simulink model "gm_sampleModel1762_5_sub"  (R2023a)
settings: Solver=VariableStepAuto  StartTime=0.0  StopTime=10.0  RelTol=1e-3
settings Model: Creator=user1  LastModifiedBy=user1
settings OptimizationCC: BlockReduction=off  ConditionallyExecuteInputs=off
settings DebuggingCC: InheritedTsInSrcMsg=none

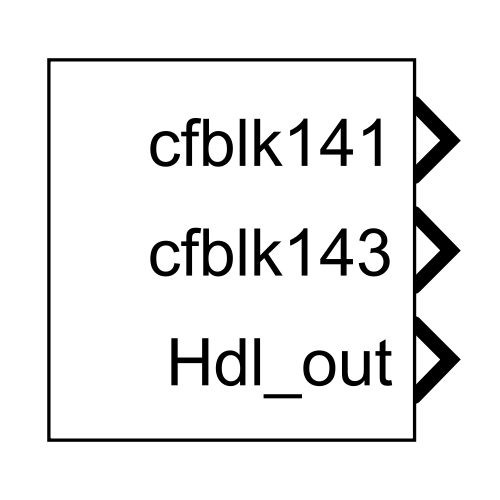
[thumbnail: Simulink's stored preview of the top-level diagram]
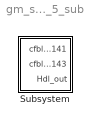
== system gm_sampleModel1762_5_sub ==
  Subsystem : Subsystem

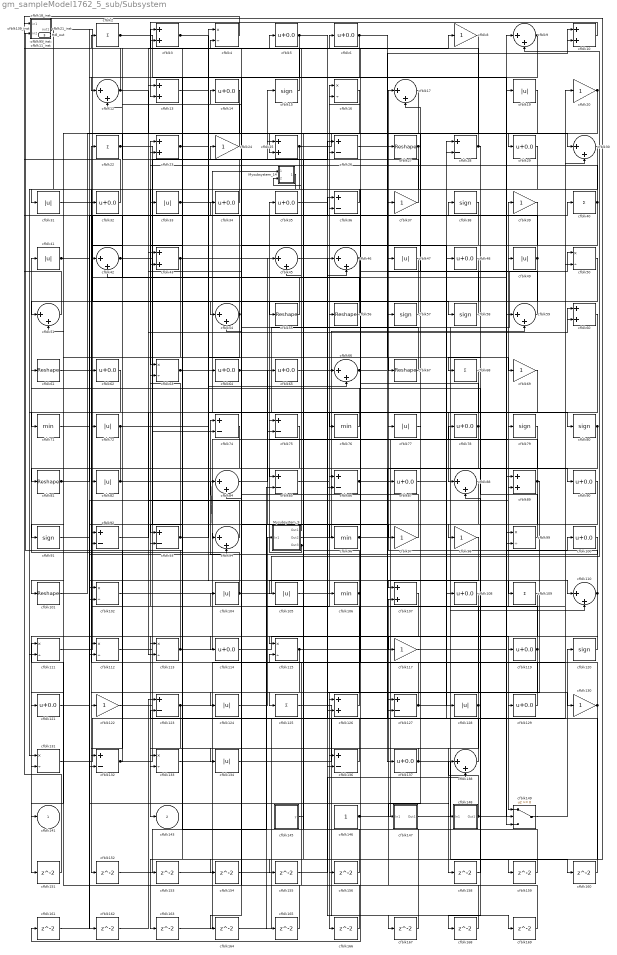
== system gm_sampleModel1762_5_sub/Subsystem ==
  Mysubsystem_14 : Subsystem
  Mysubsystem_9 : Subsystem
  cfblk{3,10,13,23,25,43,60,89,107,126} (10 alike) : Sum  OutDataTypeStr=uint8
  cfblk{5..6,14,29,32,34..35,48,62,64..65,78,87,90,100,108,114,119,121,129,137} (21 alike) : Bias  Bias=0.0  SaturateOnIntegerOverflow=off
  cfblk{27,55..56,61,67,81,101} (7 alike) : Reshape
  cfblk{4,16,50,63,99,102,111..113,115,131,133} (12 alike) : Product  Inputs=*/  OutDataTypeStr=uint8  RndMeth=Zero  SaturateOnIntegerOverflow=on
  cfblk103_inst : Subsystem
  cfblk{19,31,33,41,47,49,72,77,82,104..105,124,128,134} (14 alike) : Abs  OutDataTypeStr=uint8  SaturateOnIntegerOverflow=off
  cfblk{71,76,96,106} (4 alike) : MinMax  OutDataTypeStr=uint8
  cfblk{2,22,40,68,109,125} (6 alike) : Sum  Inputs=+  OutDataTypeStr=uint8
  cfblk{9,12,17,30,42,45..46,51,54,59,66,84,88,94,110,138} (16 alike) : Sum  Inputs=|++  OutDataTypeStr=uint8
  cfblk{8,20,24,37,39,69,97..98,117,122,130} (11 alike) : Gain  OutDataTypeStr=uint8
  cfblk11_inst : Subsystem
  cfblk{15,38,57..58,79..80,91,120} (8 alike) : Signum
  cfblk{26,28,36,74..75,85..86,92..93,123,127,132,136} (13 alike) : Sum  Inputs=+-  OutDataTypeStr=uint8
  cfblk139_inst : Subsystem
  cfblk145 : Subsystem  mask(Counter Free-Running){NumBits=double(16), tsamp=double(-1)}
      mask prompts: NumBits "Simulink:masks:NumberOfBits_MP"; tsamp "Simulink:masks:SampleTime_MP"
      mask help: Simulink:masks:CounterFreeRunning_MD
  cfblk146 : Constant  OutDataTypeStr=uint8  SampleTime=-1
  cfblk147 : Subsystem
  cfblk148 : Subsystem
  cfblk149 : Switch  OutDataTypeStr=uint8  SaturateOnIntegerOverflow=off  InputSameDT=off
  cfblk{151..156,158..169} (18 alike) : Delay  SampleTime=1
  cfblk18_inst : Subsystem
  cfblk21_inst : Subsystem
  cfblk95_inst : Subsystem
  cfblk141 : Outport  OutDataTypeStr=uint8  SampleTime=1  VectorParamsAs1DForOutWhenUnconnected=off
  cfblk143 : Outport  Port=2  OutDataTypeStr=uint8  SampleTime=1  VectorParamsAs1DForOutWhenUnconnected=off
  Hdl_out : Outport  Port=3  OutDataTypeStr=uint8  SampleTime=1
  wires:
  Mysubsystem_14/1(Out1) -> cfblk152/1
  Mysubsystem_9/1(Out1) -> cfblk45/2
  Mysubsystem_9/2(Out2) -> cfblk59/2
  Mysubsystem_9/3(Out3) -> cfblk4/2, cfblk24/1
  cfblk10/1 -> cfblk13/2
  cfblk100/1 -> cfblk74/1
  cfblk101/1 -> cfblk25/2
  cfblk102/1 -> cfblk17/1
  cfblk103_inst/1(out1) -> cfblk58/1, Hdl_out/1
  cfblk104/1 -> cfblk9/2, cfblk84/2, cfblk41/1
  cfblk105/1 -> cfblk16/1
  cfblk106/1 -> cfblk42/2, cfblk166/1
  cfblk107/1 -> cfblk143/1
  cfblk108/1 -> cfblk161/1
  cfblk109/1 -> cfblk149/1
  cfblk11_inst/1(out1) -> cfblk159/1
  cfblk110/1 -> cfblk77/1, cfblk151/1, cfblk131/2
  cfblk111/1 -> cfblk35/1
  cfblk112/1 -> cfblk74/2
  cfblk113/1 -> cfblk36/2, cfblk139_inst/2(in2)
  cfblk114/1 -> cfblk119/1
  cfblk115/1 -> cfblk28/2, cfblk122/1
  cfblk117/1 -> cfblk19/1
  cfblk119/1 -> cfblk23/1, cfblk126/1, cfblk39/1, cfblk125/1
  cfblk12/1 -> cfblk95_inst/1(in1), cfblk30/1
  cfblk120/1 -> cfblk114/1
  cfblk121/1 -> cfblk89/2
  cfblk122/1 -> cfblk37/1
  cfblk123/1 -> cfblk48/1, cfblk133/2
  cfblk124/1 -> cfblk106/1
  cfblk125/1 -> cfblk167/1
  cfblk126/1 -> cfblk22/1
  cfblk127/1 -> cfblk92/1, cfblk50/1
  cfblk128/1 -> cfblk158/1, cfblk156/1, Mysubsystem_9/1(In1)
  cfblk129/1 -> cfblk14/1
  cfblk13/1 -> cfblk110/1
  cfblk130/1 -> cfblk163/1, cfblk16/2
  cfblk131/1 -> cfblk107/2
  cfblk132/1 -> cfblk92/2, cfblk87/1, cfblk38/1
  cfblk133/1 -> cfblk57/1
  cfblk134/1 -> cfblk27/1
  cfblk136/1 -> cfblk123/2
  cfblk137/1 -> cfblk160/1, cfblk133/1
  cfblk138/1 -> cfblk104/1
  cfblk139_inst/1(out1) -> cfblk162/1
  cfblk14/1 -> cfblk51/2
  cfblk145/1(y) -> cfblk75/1
  cfblk146/1 -> cfblk59/1, cfblk20/1
  cfblk147/1(Out1) -> cfblk110/2
  cfblk148/1(Out1) -> cfblk138/1, cfblk100/1
  cfblk149/1 -> cfblk120/1
  cfblk15/1 -> cfblk5/1
  cfblk151/1 -> cfblk18_inst/2(in2)
  cfblk152/1 -> cfblk85/2
  cfblk153/1 -> cfblk50/2
  cfblk154/1 -> cfblk46/1
  cfblk155/1 -> cfblk138/2
  cfblk156/1 -> cfblk25/1
  cfblk158/1 -> cfblk88/2
  cfblk159/1 -> cfblk3/1
  cfblk16/1 -> cfblk132/1
  cfblk160/1 -> cfblk28/1
  cfblk161/1 -> cfblk102/1
  cfblk162/1 -> cfblk123/1
  cfblk163/1 -> cfblk99/2
  cfblk164/1 -> cfblk30/2
  cfblk165/1 -> cfblk54/2
  cfblk166/1 -> cfblk115/2
  cfblk167/1 -> cfblk93/2
  cfblk168/1 -> cfblk127/1
  cfblk169/1 -> cfblk111/1
  cfblk17/1 -> cfblk115/1
  cfblk18_inst/1(out1) -> cfblk66/1
  cfblk19/1 -> cfblk147/1(In1)
  cfblk2/1 -> cfblk89/1, cfblk6/1
  cfblk20/1 -> cfblk72/1, cfblk42/1
  cfblk21_inst/1(out1) -> cfblk131/1
  cfblk22/1 -> cfblk8/1, cfblk165/1
  cfblk23/1 -> cfblk66/2, cfblk76/1
  cfblk24/1 -> cfblk21_inst/1(in1)
  cfblk25/1 -> cfblk29/1, cfblk71/1
  cfblk26/1 -> cfblk69/1
  cfblk27/1 -> cfblk136/1, cfblk63/1
  cfblk28/1 -> cfblk95_inst/2(in2), cfblk68/1
  cfblk29/1 -> cfblk153/1
  cfblk3/1 -> cfblk67/1, cfblk45/1
  cfblk30/1 -> cfblk124/1
  cfblk31/1 -> cfblk108/1
  cfblk32/1 -> cfblk11_inst/2(in2)
  cfblk33/1 -> cfblk136/2, Mysubsystem_14/1(In1)
  cfblk34/1 -> cfblk2/1
  cfblk35/1 -> cfblk46/2
  cfblk36/1 -> cfblk31/1
  cfblk37/1 -> cfblk12/2
  cfblk38/1 -> cfblk155/1
  cfblk39/1 -> cfblk168/1
  cfblk4/1 -> cfblk139_inst/1(in1)
  cfblk40/1 -> cfblk23/2, cfblk126/2, cfblk164/1
  cfblk41/1 -> cfblk94/2, cfblk34/1
  cfblk42/1 -> cfblk15/1, cfblk40/1
  cfblk43/1 -> cfblk137/1, cfblk132/2
  cfblk45/1 -> cfblk80/1
  cfblk46/1 -> cfblk93/1, cfblk75/2
  cfblk47/1 -> cfblk121/1
  cfblk48/1 -> cfblk91/1
  cfblk49/1 -> cfblk54/1, cfblk26/2, cfblk103_inst/1(in1)
  cfblk5/1 -> cfblk130/1, cfblk113/1
  cfblk50/1 -> cfblk55/1
  cfblk51/1 -> cfblk21_inst/2(in2)
  cfblk54/1 -> cfblk103_inst/2(in2), cfblk101/1
  cfblk55/1 -> cfblk33/1
  cfblk56/1 -> cfblk32/1
  cfblk57/1 -> cfblk51/1
  cfblk58/1 -> cfblk17/2
  cfblk59/1 -> cfblk3/2
  cfblk6/1 -> cfblk47/1, cfblk12/1
  cfblk60/1 -> cfblk112/1
  cfblk61/1 -> cfblk9/1
  cfblk62/1 -> cfblk111/2
  cfblk63/1 -> cfblk149/2, cfblk99/1
  cfblk64/1 -> cfblk86/2, cfblk10/1
  cfblk65/1 -> cfblk169/1
  cfblk66/1 -> cfblk60/1, cfblk10/2
  cfblk67/1 -> cfblk11_inst/1(in1)
  cfblk68/1 -> cfblk88/1
  cfblk69/1 -> cfblk113/2
  cfblk71/1 -> cfblk62/1
  cfblk72/1 -> cfblk64/1, cfblk60/2, cfblk112/2
  cfblk74/1 -> cfblk141/1
  cfblk75/1 -> cfblk82/1
  cfblk76/1 -> cfblk4/1
  cfblk77/1 -> cfblk107/1
  cfblk78/1 -> cfblk18_inst/1(in1), cfblk127/2
  cfblk79/1 -> cfblk98/1
  cfblk8/1 -> cfblk43/2
  cfblk80/1 -> cfblk85/1, cfblk149/3
  cfblk81/1 -> cfblk36/1, cfblk109/1
  cfblk82/1 -> cfblk94/1, cfblk81/1
  cfblk84/1 -> cfblk65/1
  cfblk85/1 -> cfblk86/1
  cfblk86/1 -> cfblk90/1, cfblk78/1
  cfblk87/1 -> cfblk128/1
  cfblk88/1 -> cfblk105/1
  cfblk89/1 -> cfblk129/1, Mysubsystem_14/2(In2), cfblk96/1
  cfblk9/1 -> cfblk154/1, cfblk102/2
  cfblk90/1 -> cfblk134/1
  cfblk91/1 -> cfblk148/1(In1)
  cfblk92/1 -> cfblk56/1
  cfblk93/1 -> cfblk84/1, cfblk26/1, cfblk63/2
  cfblk94/1 -> cfblk13/1
  cfblk95_inst/1(out1) -> cfblk97/1
  cfblk96/1 -> cfblk79/1, cfblk49/1
  cfblk97/1 -> cfblk43/1
  cfblk98/1 -> cfblk117/1
  cfblk99/1 -> cfblk61/1

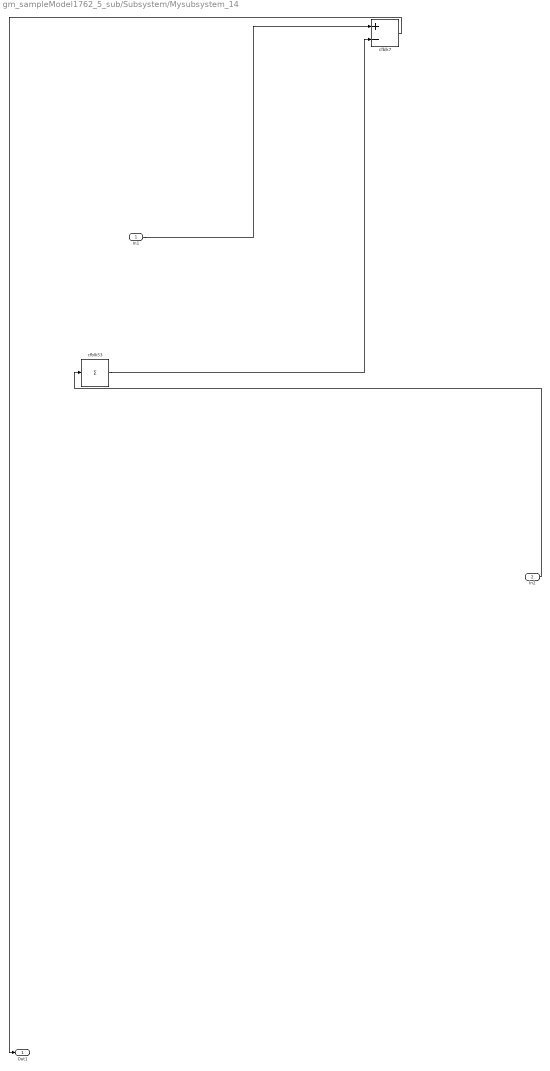
== system gm_sampleModel1762_5_sub/Subsystem/Mysubsystem_14 ==
  In1 : Inport  OutDataTypeStr=uint8  PortDimensions=1  SampleTime=1
  In2 : Inport  Port=2  OutDataTypeStr=uint8  PortDimensions=1  SampleTime=1
  cfblk53 : Sum  Inputs=+
  cfblk7 : Sum  Inputs=+-
  Out1 : Outport  SampleTime=1
  wires:
  In1/1 -> cfblk7/1
  In2/1 -> cfblk53/1
  cfblk53/1 -> cfblk7/2
  cfblk7/1 -> Out1/1

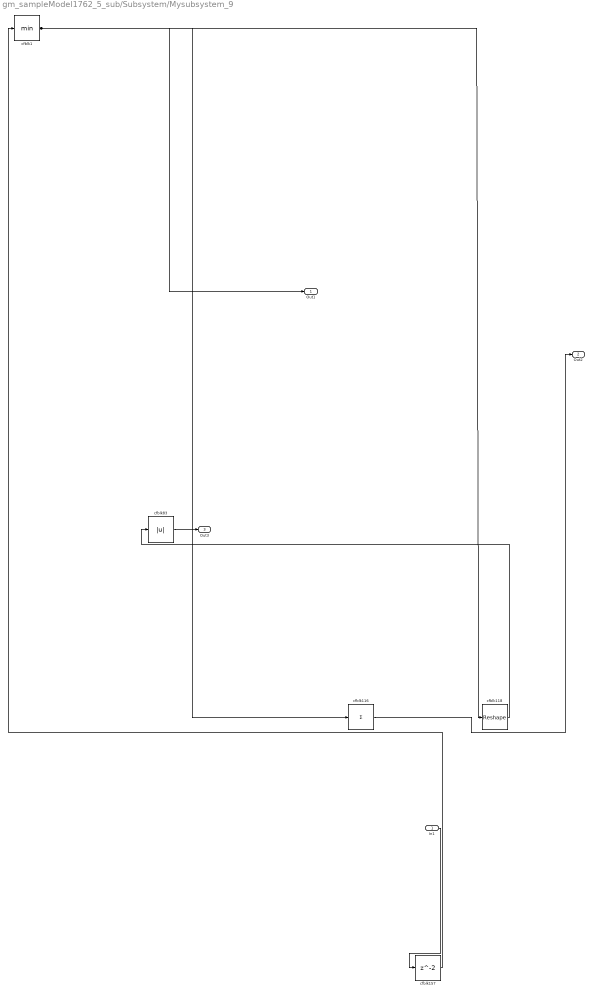
== system gm_sampleModel1762_5_sub/Subsystem/Mysubsystem_9 ==
  In1 : Inport  OutDataTypeStr=uint8  PortDimensions=1  SampleTime=1
  cfblk1 : MinMax
  cfblk116 : Sum  Inputs=+
  cfblk118 : Reshape
  cfblk157 : Delay  SampleTime=1
  cfblk83 : Abs  SaturateOnIntegerOverflow=off
  Out1 : Outport  SampleTime=1
  Out2 : Outport  Port=2  SampleTime=1
  Out3 : Outport  Port=3  SampleTime=1
  wires:
  In1/1 -> cfblk157/1
  cfblk1/1 -> cfblk118/1, Out1/1, cfblk116/1
  cfblk116/1 -> Out2/1
  cfblk118/1 -> cfblk83/1
  cfblk157/1 -> cfblk1/1
  cfblk83/1 -> Out3/1

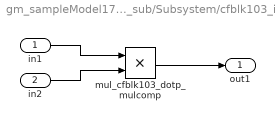
== system gm_sampleModel1762_5_sub/Subsystem/cfblk103_inst ==
  in1 : Inport  OutDataTypeStr=uint8  SampleTime=1
  in2 : Inport  Port=2  OutDataTypeStr=uint8  SampleTime=1
  mul_cfblk103_dotp_mulcomp : Product  Inputs=**  OutDataTypeStr=uint8  SampleTime=1
  out1 : Outport  OutDataTypeStr=uint8  SampleTime=1
  wires:
  in1/1 -> mul_cfblk103_dotp_mulcomp/1
  in2/1 -> mul_cfblk103_dotp_mulcomp/2
  mul_cfblk103_dotp_mulcomp/1 -> out1/1

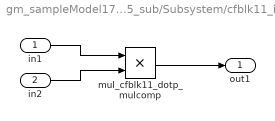
== system gm_sampleModel1762_5_sub/Subsystem/cfblk11_inst ==
  in1 : Inport  OutDataTypeStr=uint8  SampleTime=1
  in2 : Inport  Port=2  OutDataTypeStr=uint8  SampleTime=1
  mul_cfblk11_dotp_mulcomp : Product  Inputs=**  OutDataTypeStr=uint8  SampleTime=1
  out1 : Outport  OutDataTypeStr=uint8  SampleTime=1
  wires:
  in1/1 -> mul_cfblk11_dotp_mulcomp/1
  in2/1 -> mul_cfblk11_dotp_mulcomp/2
  mul_cfblk11_dotp_mulcomp/1 -> out1/1

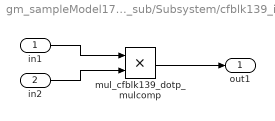
== system gm_sampleModel1762_5_sub/Subsystem/cfblk139_inst ==
  in1 : Inport  OutDataTypeStr=uint8  SampleTime=1
  in2 : Inport  Port=2  OutDataTypeStr=uint8  SampleTime=1
  mul_cfblk139_dotp_mulcomp : Product  Inputs=**  OutDataTypeStr=uint8  SampleTime=1
  out1 : Outport  OutDataTypeStr=uint8  SampleTime=1
  wires:
  in1/1 -> mul_cfblk139_dotp_mulcomp/1
  in2/1 -> mul_cfblk139_dotp_mulcomp/2
  mul_cfblk139_dotp_mulcomp/1 -> out1/1

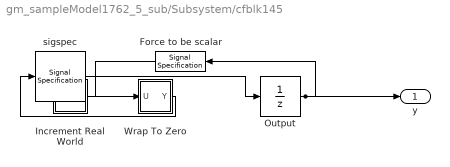
== system gm_sampleModel1762_5_sub/Subsystem/cfblk145 ==
  Force to be scalar : SignalSpecification  DisableCoverage=on  Dimensions=1
  Increment Real World : Subsystem  mask(Real World Value Increment){}
      mask help: Simulink:masks:RealWorldValueIncrement_MD
      mask Display: disp('V++')
  Output : UnitDelay  InitialCondition=0.0  SampleTime=tsamp  HasFrameUpgradeWarning=on
  Wrap To Zero : Subsystem  mask(Wrap To Zero){Threshold=double(65535)}
      mask prompts: Threshold "Simulink:masks:Threshold_MP"
      mask help: Simulink:masks:WrapToZero_MD
  sigspec : SignalSpecification  OutDataTypeStr=uint16  Dimensions=1
  y : Outport  SampleTime=1
  wires:
  Force to be scalar/1 -> Increment Real World/1(u)
  Increment Real World/1(y) -> Wrap To Zero/1(U)
  Output/1 -> Force to be scalar/1, y/1
  Wrap To Zero/1(Y) -> sigspec/1
  sigspec/1 -> Output/1

== system gm_sampleModel1762_5_sub/Subsystem/cfblk147 ==
  In1 : Inport  OutDataTypeStr=uint8  PortDimensions=1  SampleTime=1
  Out1 : Outport  SampleTime=1
  wires:
  In1/1 -> Out1/1

== system gm_sampleModel1762_5_sub/Subsystem/cfblk148 ==
  In1 : Inport  OutDataTypeStr=uint8  PortDimensions=1  SampleTime=1
  Out1 : Outport  SampleTime=1
  wires:
  In1/1 -> Out1/1

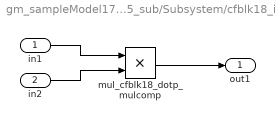
== system gm_sampleModel1762_5_sub/Subsystem/cfblk18_inst ==
  in1 : Inport  OutDataTypeStr=uint8  SampleTime=1
  in2 : Inport  Port=2  OutDataTypeStr=uint8  SampleTime=1
  mul_cfblk18_dotp_mulcomp : Product  Inputs=**  OutDataTypeStr=uint8  SampleTime=1
  out1 : Outport  OutDataTypeStr=uint8  SampleTime=1
  wires:
  in1/1 -> mul_cfblk18_dotp_mulcomp/1
  in2/1 -> mul_cfblk18_dotp_mulcomp/2
  mul_cfblk18_dotp_mulcomp/1 -> out1/1

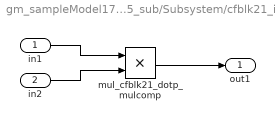
== system gm_sampleModel1762_5_sub/Subsystem/cfblk21_inst ==
  in1 : Inport  OutDataTypeStr=uint8  SampleTime=1
  in2 : Inport  Port=2  OutDataTypeStr=uint8  SampleTime=1
  mul_cfblk21_dotp_mulcomp : Product  Inputs=**  OutDataTypeStr=uint8  SampleTime=1
  out1 : Outport  OutDataTypeStr=uint8  SampleTime=1
  wires:
  in1/1 -> mul_cfblk21_dotp_mulcomp/1
  in2/1 -> mul_cfblk21_dotp_mulcomp/2
  mul_cfblk21_dotp_mulcomp/1 -> out1/1

== system gm_sampleModel1762_5_sub/Subsystem/cfblk95_inst ==
  in1 : Inport  OutDataTypeStr=uint8  SampleTime=1
  in2 : Inport  Port=2  OutDataTypeStr=uint8  SampleTime=1
  mul_cfblk95_dotp_mulcomp : Product  Inputs=**  OutDataTypeStr=uint8  SampleTime=1
  out1 : Outport  OutDataTypeStr=uint8  SampleTime=1
  wires:
  in1/1 -> mul_cfblk95_dotp_mulcomp/1
  in2/1 -> mul_cfblk95_dotp_mulcomp/2
  mul_cfblk95_dotp_mulcomp/1 -> out1/1

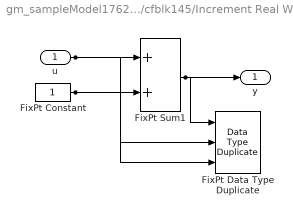
== system gm_sampleModel1762_5_sub/Subsystem/cfblk145/Increment Real World ==
  u : Inport  OutDataTypeStr=uint16  SampleTime=1
  FixPt Constant : Constant  DisableCoverage=on  OutDataTypeStr=Inherit: Inherit via back propagation  SampleTime=-1
  FixPt Data Type Duplicate : DataTypeDuplicate  DisableCoverage=on  NumInputPorts=3
  FixPt Sum1 : Sum  InputSameDT=on  OutDataTypeStr=Inherit: Inherit via back propagation  LockScale=on
  y : Outport  SampleTime=1
  wires:
  u/1 -> FixPt Sum1/1, FixPt Data Type Duplicate/2
  FixPt Constant/1 -> FixPt Sum1/2, FixPt Data Type Duplicate/3
  FixPt Sum1/1 -> FixPt Data Type Duplicate/1, y/1

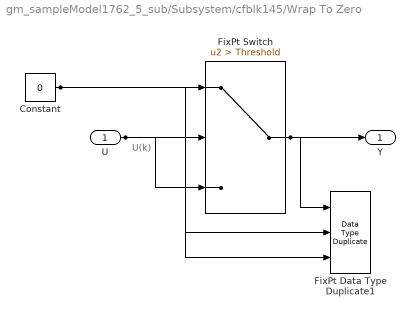
== system gm_sampleModel1762_5_sub/Subsystem/cfblk145/Wrap To Zero ==
  note: U(k)
  U : Inport  OutDataTypeStr=uint16  SampleTime=1
  Constant : Constant  DisableCoverage=on  Value=0  OutDataTypeStr=Inherit: Inherit via back propagation  SampleTime=-1
  FixPt Data Type Duplicate1 : DataTypeDuplicate  DisableCoverage=on  NumInputPorts=3
  FixPt Switch : Switch  Criteria=u2 > Threshold  Threshold=Threshold  OutDataTypeStr=Inherit: Inherit via back propagation  ZeroCross=off  SaturateOnIntegerOverflow=off  InputSameDT=off
  Y : Outport  SampleTime=1
  wires:
  U/1 -> FixPt Switch/3, FixPt Switch/2, FixPt Data Type Duplicate1/2
  Constant/1 -> FixPt Switch/1, FixPt Data Type Duplicate1/3
  FixPt Switch/1 -> FixPt Data Type Duplicate1/1, Y/1
